simulink library "ActivationContainerEnabled"  (R2017b)
settings: Solver=VariableStepAuto  StartTime=0.0  StopTime=10.0  RelTol=1e-3
settings Model: Creator=Beni  LastModifiedBy=Beni

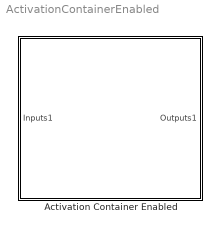
== system ActivationContainerEnabled ==
  Activation Container Enabled : Subsystem  mask(BlockActivationEnabled){Status0=Active, Activation0=1, Status1=Inactive, Activation1=0, Status2=Inactive, Activation2=0, Status3=Inactive, Activation3=0, Status4=Inactive, Activation4=0, Status5=Inactive, Activation5=0, Status6=Inactive, Activation6=0, Status7=Inactive, Activation7=0, Status8=Inactive, Activation8=0, Status9=Inactive, Activation9=0}
      mask prompts: Status0 "Activity status of "Enabled Subsystem0":"; Activation0 "Invisible Help Variable"; Status1 "Activity status of "Enabled Subsystem1":"; Activation1 "Invisible Help Variable"; Status2 "Activity status of "Enabled Subsystem2":"; Activation2 "Invisible Help Variable"; Status3 "Activity status of "Enabled Subsystem3":"; Activation3 "Invisible Help Variable"; Status4 "Activity status of "Enabled Subsystem4":"; Activation4 "Invisible Help Variable"; Status5 "Activity status of "Enabled Subsystem5":"; Activation5 "Invisible Help Variable"; Status6 "Activity status of "Enabled Subsystem6":"; Activation6 "Invisible Help Variable"; Status7 "Activity status of "Enabled Subsystem7" [-]:"; Activation7 "Invisible Help Variable"; Status8 "Activity status of "Enabled Subsystem8" [-]:"; Activation8 "Invisible Help Variable"; Status9 "Activity status of "Enabled Subsystem9" [-]:"; Activation9 "Invisible Help Variable"
      mask help:
      | <Author> Benedikt Taiber </Author>
      | <Date> 25/09/2018 </Date>
      |
      | <Description>
      | This block can contain up to ten enabled subsystems, that can be activated or deactivated for the simulation, depending on the user's input within the mask dialog. New subsystems can be added or already existing subsystems deleted by clicking the corresponding buttons on the mask dialog. The subsystems can also be de-/activated programmatically by setting the parameters "ActivationX" and "StatusX" to the corresponding "SubsystemX" to " '1/0' " and " 'Active/Inactive' ".
      | </Description>
      mask init:
      | init_activation_container();
      settings: OpenFcn=|
      | set_param(gcb,'LinkStatus','none');
      | init_activation_container();
      | open_system(gcb,'mask');
      mask Help:
      | <Parameters>
      | Activity status of "EnabledSubsystemX" [-]:
      | 	<Active, Inactive>
      | </Parameters>
      | 
      | <Inputs>
      | Depending on content of subsystem
      | </Inputs>
      | 
      | <Outputs>
      | Depending on content of subsystem
      | </Outputs>
      mask TypeOptions Status0: Active | Inactive
      mask Callback Status0:
      | if strcmp(get_param(gcb,'Status0'),'Active')
      |     set_param(gcb,'Activation0','1');
      | elseif strcmp(get_param(gcb,'Status0'),'Inactive')
      |     set_param(gcb,'Activation0','0');
      | end
      mask TypeOptions Status1: Active | Inactive
      mask Callback Status1:
      | if strcmp(get_param(gcb,'Status1'),'Active')
      |     set_param(gcb,'Activation1','1');
      | elseif strcmp(get_param(gcb,'Status1'),'Inactive')
      |     set_param(gcb,'Activation1','0');
      | end
      mask TypeOptions Status2: Active | Inactive
      mask Callback Status2:
      | if strcmp(get_param(gcb,'Status2'),'Active')
      |     set_param(gcb,'Activation2','1');
      | elseif strcmp(get_param(gcb,'Status2'),'Inactive')
      |     set_param(gcb,'Activation2','0');
      | end
      mask TypeOptions Status3: Active | Inactive
      mask Callback Status3:
      | if strcmp(get_param(gcb,'Status3'),'Active')
      |     set_param(gcb,'Activation3','1');
      | elseif strcmp(get_param(gcb,'Status3'),'Inactive')
      |     set_param(gcb,'Activation3','0');
      | end
      mask TypeOptions Status4: Active | Inactive
      mask Callback Status4:
      | if strcmp(get_param(gcb,'Status4'),'Active')
      |     set_param(gcb,'Activation4','1');
      | elseif strcmp(get_param(gcb,'Status4'),'Inactive')
      |     set_param(gcb,'Activation4','0');
      | end
      mask TypeOptions Status5: Active | Inactive
      mask Callback Status5:
      | if strcmp(get_param(gcb,'Status5'),'Active')
      |     set_param(gcb,'Activation5','1');
      | elseif strcmp(get_param(gcb,'Status5'),'Inactive')
      |     set_param(gcb,'Activation5','0');
      | end
      mask TypeOptions Status6: Active | Inactive
      mask Callback Status6:
      | if strcmp(get_param(gcb,'Status6'),'Active')
      |     set_param(gcb,'Activation6','1');
      | elseif strcmp(get_param(gcb,'Status6'),'Inactive')
      |     set_param(gcb,'Activation6','0');
      | end
      mask TypeOptions Status7: Active | Inactive
      mask Callback Status7:
      | if strcmp(get_param(gcb,'Status7'),'Active')
      |     set_param(gcb,'Activation7','1');
      | elseif strcmp(get_param(gcb,'Status7'),'Inactive')
      |     set_param(gcb,'Activation7','0');
      | end
      mask TypeOptions Status8: Active | Inactive
      mask Callback Status8:
      | if strcmp(get_param(gcb,'Status8'),'Active')
      |     set_param(gcb,'Activation8','1');
      | elseif strcmp(get_param(gcb,'Status8'),'Inactive')
      |     set_param(gcb,'Activation8','0');
      | end
      mask TypeOptions Status9: Active | Inactive
      mask Callback Status9:
      | if strcmp(get_param(gcb,'Status9'),'Active')
      |     set_param(gcb,'Activation9','1');
      | elseif strcmp(get_param(gcb,'Status9'),'Inactive')
      |     set_param(gcb,'Activation9','0');
      | end
      mask DialogControl Container14 Prompt: Documentation:
      mask DialogControl Control14 Prompt: %<MaskHelp>
      mask DialogControl Container0 Prompt: "Activation0":
      mask DialogControl Delete0 Prompt: Delete Subsystem
      mask DialogControl Delete0 Callback:
      | index = 0;
      | init_delete_button(index);
      | clear index
      mask DialogControl Container1 Prompt: "Activation1":
      mask DialogControl Delete1 Prompt: Delete Subsystem
      mask DialogControl Delete1 Callback:
      | index = 1;
      | init_delete_button(index);
      | clear index;
      mask DialogControl Container2 Prompt: "Activation2":
      mask DialogControl Delete2 Prompt: Delete Subsystem
      mask DialogControl Delete2 Callback:
      | index = 2;
      | init_delete_button(index);
      | clear index
      mask DialogControl Container3 Prompt: "Activation3":
      mask DialogControl Delete3 Prompt: Delete Subsystem
      mask DialogControl Delete3 Callback:
      | index = 3;
      | init_delete_button(index);
      | clear index
      mask DialogControl Container4 Prompt: "Activation4":
      mask DialogControl Delete4 Prompt: Delete Subsystem
      mask DialogControl Delete4 Callback:
      | index = 4;
      | init_delete_button(index);
      | clear index
      mask DialogControl Container5 Prompt: "Activation5":
      mask DialogControl Delete5 Prompt: Delete Subsystem
      mask DialogControl Delete5 Callback:
      | index = 5;
      | init_delete_button(index);
      | clear index
      mask DialogControl Container6 Prompt: "Activation6":
      mask DialogControl Delete6 Prompt: Delete Subsystem
      mask DialogControl Delete6 Callback:
      | index = 6;
      | init_delete_button(index);
      | clear index
      mask DialogControl Container7 Prompt: "Activation7":
      mask DialogControl Delete7 Prompt: Delete Subsystem
      mask DialogControl Delete7 Callback:
      | index = 7;
      | init_delete_button(index);
      | clear index
      mask DialogControl Container8 Prompt: "Activation8":
      mask DialogControl Delete8 Prompt: Delete Subsystem
      mask DialogControl Delete8 Callback:
      | index = 8;
      | init_delete_button(index);
      | clear index
      mask DialogControl Container9 Prompt: "Activation9":
      mask DialogControl Delete9 Prompt: Delete Subsystem
      mask DialogControl Delete9 Callback:
      | index = 9;
      | init_delete_button(index);
      | clear index
      mask DialogControl ContainerControls Prompt: Controls:
      mask DialogControl new_system Prompt: Create new subsystem
      mask DialogControl new_system Callback:
      | init_new_subsystem();
      | init_activation_container();
      mask DialogControl check_system Prompt: Look under mask
      mask DialogControl check_system Callback: open_system(gcb,'force')

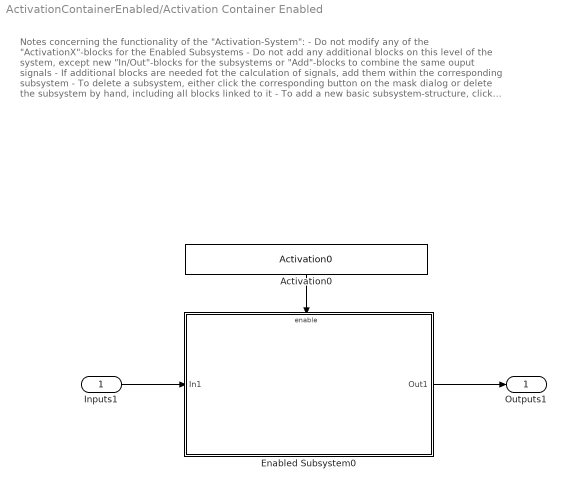
== system ActivationContainerEnabled/Activation Container Enabled ==
  note: Notes concerning the functionality of the "Activation-System":
      |
      | - Do not modify any of the "ActivationX"-blocks for the Enabled Subsystems
      | - Do not add any additional blocks on this level of the system, except new "In/Out"-blocks for
      |   the subsystems or "Add"-blocks to combine the same ouput signals
      | - If additional blocks are needed fot the calculation of signals, add them within the
      |   corresponding subsystem
      | - To delete a subsystem, either click the corresponding button on the mask dialog or delete
      |   the subsystem by hand, including all blocks linked to it
      | - To add a new basic subsystem-structure, click the button on the mask dialog
  Inputs1 : Inport
  Activation0 : Constant  Value=Activation0
  Enabled Subsystem0 : Subsystem  TreatAsAtomicUnit=on
  Outputs1 : Outport
  wires:
  Inputs1/1 -> Enabled Subsystem0/1(In1)
  Enabled Subsystem0/1(Out1) -> Outputs1/1
  Activation0/1 -> Enabled Subsystem0/Enable

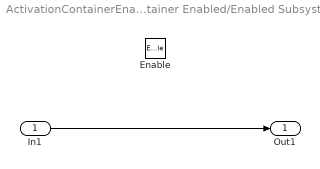
== system ActivationContainerEnabled/Activation Container Enabled/Enabled Subsystem0 ==
  In1 : Inport
  Enable : EnablePort
  Out1 : Outport
  wires:
  In1/1 -> Out1/1
